simulink model "untitled1"  (R2021a)
settings: Solver=VariableStepAuto  StartTime=0.0  StopTime=10.0  RelTol=1e-3
settings Model: Creator=ewlee  LastModifiedBy=ewlee

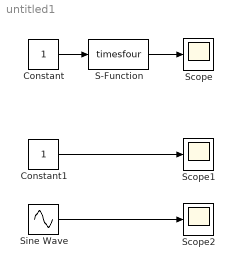
== system untitled1 ==
  Constant : Constant
  Constant1 : Constant
  S-Function : S-Function  FunctionName=timesfour  SFunctionDeploymentMode=off  EnableBusSupport=off
  Scope : Scope
  Scope1 : Scope
  Scope2 : Scope
  Sine Wave : Sin  SampleTime=0
  wires:
  Constant/1 -> S-Function/1
  S-Function/1 -> Scope/1
  Constant1/1 -> Scope1/1
  Sine Wave/1 -> Scope2/1
